simulink model "simulink_ros"  (R2022b)
settings: Solver=FixedStepAuto  StartTime=0.0  StopTime=inf  FixedStep=0.01  RelTol=1e-3
InitFcn:
  | %INIT_COSIM
undefined symbols (not defined in the file or in its folder): nmpc_controller, setup
libraries: robotlib x5
settings Model: Creator=pico  LastModifiedBy=pico

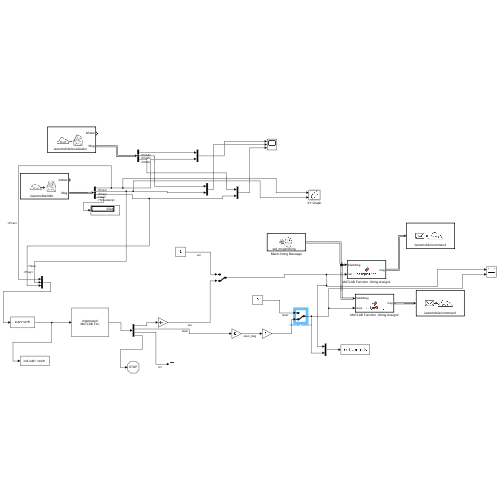
[thumbnail: Simulink's stored preview of the top-level diagram]
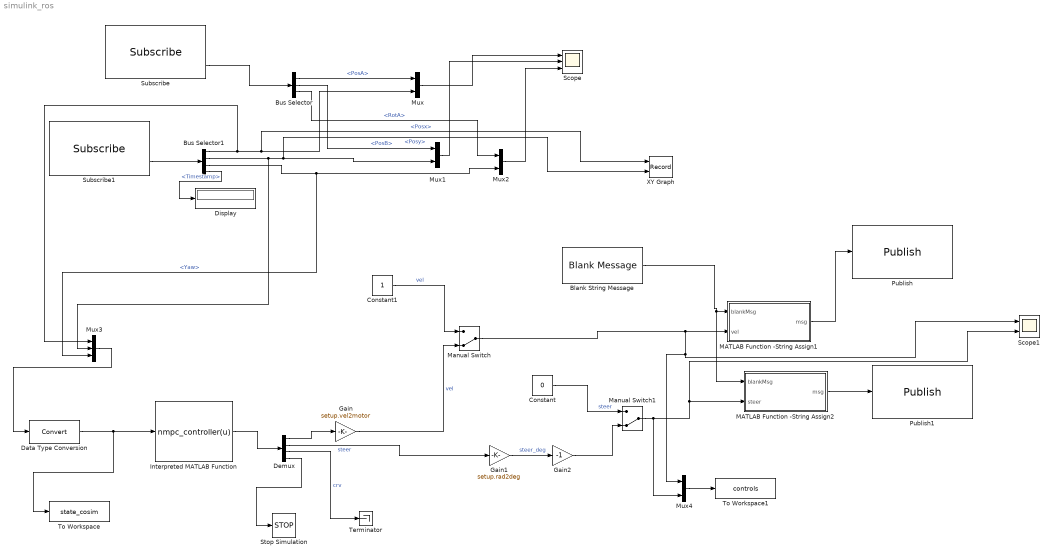
== system simulink_ros ==
  Blank String Message : robotlib/Blank Message  messageClass=Message  entityType=std_msgs/String  messageType=std_msgs/String  SampleTime=inf  legacyBusStruct=off
  Bus Selector : BusSelector  OutputSignals=PosA,PosB,RotA
  Bus Selector1 : BusSelector  OutputSignals=Posx,Posy,Yaw,Timestamp
  Constant : Constant  Value=0
  Constant1 : Constant
  Data Type Conversion : DataTypeConversion  SaturateOnIntegerOverflow=off  RndMeth=Floor
  Demux : Demux
  Display : Display
  Gain : Gain  Gain=setup.vel2motor
  Gain1 : Gain  Gain=setup.rad2deg
  Gain2 : Gain  Gain=-1
  Interpreted MATLAB Function : MATLABFcn  MATLABFcn=nmpc_controller(u)  OutputDimensions=4
  MATLAB Function -String Assign1 : MATLAB Function  TreatAsAtomicUnit=on
  MATLAB Function -String Assign2 : MATLAB Function  TreatAsAtomicUnit=on
  Manual Switch : ManualSwitch  CurrentSetting=0
  Manual Switch1 : ManualSwitch  CurrentSetting=0
  Mux{,1..2,4} (4 alike) : Mux  Inputs=2
  Mux3 : Mux  Inputs=3
  Publish : robotlib/Publish  topicSource=Select from ROS network  topic=/automobile/command  messageType=std_msgs/String  legacyBusStruct=off  messageQueueLength=1
      settings: LibrarySourceBlock=roslib/ROS/Publish
  Publish1 : robotlib/Publish  topicSource=Select from ROS network  topic=/automobile/command  messageType=std_msgs/String  legacyBusStruct=off  messageQueueLength=1
      settings: LibrarySourceBlock=roslib/ROS/Publish
  Scope : Scope  NumInputPorts=3
  Scope1 : Scope  NumInputPorts=2
  Stop Simulation : Stop
  Subscribe : robotlib/Subscribe  topicSource=Select from ROS network  topic=/automobile/localisation  messageType=utils/localisation  SampleTime=-1  legacyBusStruct=off  messageQueueLength=1
      settings: LibrarySourceBlock=roslib/ROS/Subscribe
  Subscribe1 : robotlib/Subscribe  topicSource=Select from ROS network  topic=/automobile/IMU  messageType=utils/IMU  SampleTime=-1  legacyBusStruct=off  messageQueueLength=1
      settings: LibrarySourceBlock=roslib/ROS/Subscribe
  Terminator : Terminator
  To Workspace : ToWorkspace  VariableName=state_cosim  SaveFormat=Structure With Time  SampleTime=-1
  To Workspace1 : ToWorkspace  VariableName=controls  SaveFormat=Structure With Time  SampleTime=-1
  XY Graph : Record  FileSettingsInternal="{\"entries\":[{\"content\":{\"excelSettings\":{\"content\":{},\"type\":\"Streamout.ExcelSettings\"}},\"type\":\"Streamout.FileSettingStorage\",\"uuid\":\"66a75b85-4887-46d6-b016-73f79b331a3a\"}],\"packageUris\":[\"http://schema.mathworks.com/mf0/streamout_blocks/R2020a\"],\"version\":\"1.0\"}"  Layout=[1 1]  SignalsInternal="{\"entries\":[{\"content\":{\"signals\":[{\"content\":{\"blockPath\":[\"simulink_ros/XY Graph\"],\"channel\":[],\"dimensions\":[1],\"domain\":\"simulink_ros/XY Graph\",\"lineColor\":\"#a2142f\",\"plots\":[1],\"port\":1,\"sid\":[\"\"],\"signalID\":6347,\"signalName\":\"<Posx>\"},\"type\":\"RecordBlkView.Signal\",\"uuid\":\"b4b6075f-ac59-459d-b2ee-449fad9a718f\"},{\"content\":{\"blockPath\":[\"simulink_ros/XY Graph\"],\"channel\":[],\"dimensions\":[1],\"domain\":\"simulink_ros/XY Graph\",\"lineColor\":\"#139fff\",\"plots\":[1],\"port\":2,\"sid\":[\"\"],\"signalID\":6351,\"signalName\":\"<Posy>\"},\"type\":\"RecordBlkView.Signal\",\"uuid\":\"0b41d109-86db-4643-8565-47aa51f1432c\"}]},\"type\":\"RecordBlkView.InputSignals\",\"uuid\":\"d370277d-2c24-4457-a44f-88554cabd6fe\"}],\"packageUris\":[\"http://schema.mathworks.com/mf0/streamout_blocks/R2020a\"],\"version\":\"1.0\"}"  VisualizationBindings="{\"xyplotplugin\":{\"info\":[{\"series\":[{\"bindingParametersList\":[{\"parameter\":\"X-Axis\",\"signalID\":6347,\"signalName\":\"<Posx>\"},{\"parameter\":\"Y-Axis\",\"signalID\":6351,\"signalName\":\"<Posy>\"}],\"seriesID\":53260}],\"subplotID\":1}]}}"  CompatibilityTag=XY
  wires:
  Subscribe/2 -> Bus Selector/1
  Bus Selector/1 -> Mux/1  "<PosA>"
  Blank String Message/1 -> MATLAB Function -String Assign2/1(blankMsg), MATLAB Function -String Assign1/1(blankMsg)
  MATLAB Function -String Assign1/1(msg) -> Publish/1
  MATLAB Function -String Assign2/1(msg) -> Publish1/1
  Subscribe1/2 -> Bus Selector1/1
  Mux/1 -> Scope/1
  Bus Selector/2 -> Mux1/1  "<PosB>"
  Mux1/1 -> Scope/2
  Bus Selector/3 -> Mux2/1  "<RotA>"
  Mux2/1 -> Scope/3
  Bus Selector1/4 -> Display/1  "<Timestamp>"
  Demux/1 -> Gain/1
  Bus Selector1/2 -> Mux3/2, XY Graph/2, Mux1/2  "<Posy>"
  Bus Selector1/3 -> Mux3/3, Mux2/2  "<Yaw>"
  Bus Selector1/1 -> Mux3/1, XY Graph/1, Mux/2  "<Posx>"
  Interpreted MATLAB Function/1 -> Demux/1
  Demux/2 -> Gain1/1  "steer"
  Gain/1 -> Manual Switch/2  "vel"
  Manual Switch/1 -> Mux4/1, Scope1/1, MATLAB Function -String Assign1/2(vel)
  Constant1/1 -> Manual Switch/1  "vel"
  Constant/1 -> Manual Switch1/1  "steer"
  Manual Switch1/1 -> Mux4/2, Scope1/2, MATLAB Function -String Assign2/2(steer)
  Data Type Conversion/1 -> To Workspace/1, Interpreted MATLAB Function/1
  Mux3/1 -> Data Type Conversion/1
  Demux/4 -> Stop Simulation/1
  Demux/3 -> Terminator/1  "crv"
  Gain1/1 -> Gain2/1  "steer_deg"
  Gain2/1 -> Manual Switch1/2
  Mux4/1 -> To Workspace1/1

== matlab function simulink_ros/MATLAB Function -String Assign2 ==
  data: blankMsg input; msg output Bus: SL_Bus_simulink_ros_std_msgs_String; steer input
function msg = assignString(blankMsg,steer)
% assignString - Assign a string in a ROS message
%
% MSG = assignString(blankMsg) assigns a known string value to a 
%  string field in a ROS message, and outputs the updated ROS message.
%
%  blankMsg (input): A bus for a 'std_msgs/String' message. This is 
%      used to initialize the output. 
%  msg (output): A bus for a 'std_msgs/String' message, with the Data 
%      field set to a string.

%   Copyright 2015 The MathWorks, Inc.
%#codegen

% Note: The datatype of 'msg' has been explicitly set to the appropriate 
% Simulink bus type ("Bus: SL_Bus_robotROSMessageUsageExample_std_msgs_String"). 
%
% If the model name is changed, the datatype needs to be changed as well:
%   1) Click "Edit Data" in the Editor toolstrip to open "Ports and Data Manager"
%   2) Select "msg". From the "Type" dropdown, select "--- Refresh data types ---"
%   3) Set datatype to "Bus: SL_Bus_<modelname>_std_msgs_String"
    
% stringToAssign = 'information';
steer_string = sprintf('%.1f',steer);
% "{\"action\": \"1\", \"speed\": -0.1}"
stringToAssign = ['{"action": "2", "steerAngle": ',steer_string,'}'];%['action\', '1', 'speed',u];

msg = blankMsg;

% msg (std_msgs/String) consists of
%           Data : array of type uint8
%   Data_SL_Info : struct with fields CurrentLength, ReceivedLength
strLength = length(stringToAssign);
msg.Data(1:strLength) = uint8(stringToAssign);
msg.Data_SL_Info.CurrentLength = uint32(strLength);

== matlab function simulink_ros/MATLAB Function -String Assign1 ==
  data: blankMsg input; msg output Bus: SL_Bus_simulink_ros_std_msgs_String; vel input
function msg = assignString(blankMsg,vel)
% assignString - Assign a string in a ROS message
%
% MSG = assignString(blankMsg) assigns a known string value to a 
%  string field in a ROS message, and outputs the updated ROS message.
%
%  blankMsg (input): A bus for a 'std_msgs/String' message. This is 
%      used to initialize the output. 
%  msg (output): A bus for a 'std_msgs/String' message, with the Data 
%      field set to a string.

%   Copyright 2015 The MathWorks, Inc.
%#codegen

% Note: The datatype of 'msg' has been explicitly set to the appropriate 
% Simulink bus type ("Bus: SL_Bus_robotROSMessageUsageExample_std_msgs_String"). 
%
% If the model name is changed, the datatype needs to be changed as well:
%   1) Click "Edit Data" in the Editor toolstrip to open "Ports and Data Manager"
%   2) Select "msg". From the "Type" dropdown, select "--- Refresh data types ---"
%   3) Set datatype to "Bus: SL_Bus_<modelname>_std_msgs_String"
    
thr_string = sprintf('%.1f',vel);
% "{\"action\": \"1\", \"speed\": -0.1}"
stringToAssign = ['{"action": "1", "speed": ',thr_string,'}'];%['action\', '1', 'speed',u];

msg = blankMsg;

% msg (std_msgs/String) consists of
%           Data : array of type uint8
%   Data_SL_Info : struct with fields CurrentLength, ReceivedLength
strLength = length(stringToAssign);
msg.Data(1:strLength) = uint8(stringToAssign);
msg.Data_SL_Info.CurrentLength = uint32(strLength);
